simulink library "fm_lib"  (R2014a)
settings: Solver=ode45  SolverMode=SingleTasking  StartTime=0.0  StopTime=10.0  RelTol=1e-3
(part 1 of 2)
Description:
  | PSAT Library
settings Model: ExtModeAutoUpdateStatusClock=off  Creator=fmilano  LastModifiedBy=m.shariatzadeh

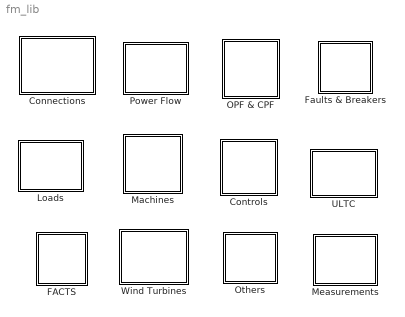
== system fm_lib ==
  Connections : Subsystem  Tag=PSATfolder  Description=Connections  mask(Bus & Connections){}
      mask init:
      | x = fm_draw('connections');
      mask Display: image(x)
  Controls : Subsystem  Tag=PSATfolder  Description=Controls
      mask init:
      | x = fm_draw('controls');
      mask Display: image(x)
  FACTS : Subsystem  Tag=PSATfolder  Description=FACTS
      mask init:
      | x = fm_draw('facts');
      mask Display: image(x)
  Faults & Breakers : Subsystem  Tag=PSATfolder  Description=Switches
      mask init:
      | x = fm_draw('fault');
      mask Display: image(x)
  Loads : Subsystem  Tag=PSATfolder  Description=Loads
      mask init:
      | x = fm_draw('loads');
      mask Display: image(x)
  Machines : Subsystem  Tag=PSATfolder  Description=Machines
      mask init:
      | x = fm_draw('machines');
      mask Display: image(x)
  Measurements : Subsystem  Tag=PSATfolder  Description=Switches
      mask init:
      | x = fm_draw('measures');
      mask Display: image(x)
  OPF & CPF : Subsystem  Tag=PSATfolder  Description=OPFandCPF
      mask init:
      | x = fm_draw('opfcpf');
      mask Display: image(x)
  Others : Subsystem  Tag=PSATfolder  Description=Others
      mask init:
      | x = fm_draw('others');
      mask Display: image(x)
  Power Flow : Subsystem  Tag=PSATfolder  Description=PowerFlow
      mask init:
      | x = fm_draw('powerflow');
      mask Display: image(x)
  ULTC : Subsystem  Tag=PSATfolder  Description=ULTC
      mask init:
      | x = fm_draw('ultc');
      mask Display: image(x)
  Wind Turbines : Subsystem  Tag=PSATfolder  Description=Controls
      mask init:
      | x = fm_draw('wind');
      mask Display: image(x)

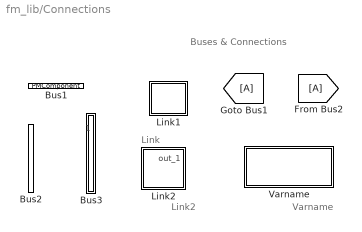
== system fm_lib/Connections ==
  note: Buses & Connections
  note: Link
  note: Link2
  note: Varname
  Bus1 : PMComponent  Tag=PSATblock  Description=Connection  PhysicalDomain=psatdomain  LeftPortType=p1  RightPortType=p1  LConnTagsString=__newl0|__newl1  RConnTagsString=__newr0  mask(Bus){in=2, out=1, p2q=400, p3_4q=[1.00  0.00], p5q=1, p6q=1}
      mask prompts: in "Number of inputs:"; out "Number of outputs:"; p2q "Voltage Rating [kV]"; p3_4q "Voltage initial guess [p.u.  rad]"; p5q "Area number"; p6q "Region number"
      mask help: Bus block.
      mask init:
      | fm_inout
      mask Callback p5q: fm_block
      mask Display: plot([0 1 1 0 0],[0 0 1 1 0])
  Bus2 : PMComponent  Tag=PSATblock  Description=Connection  PhysicalDomain=psatdomain  LeftPortType=p1  RightPortType=p1  LConnTagsString=__newl0|__newl1|__newl2  RConnTagsString=__newr0|__newr1  mask(Bus){in=3, out=2, p2q=400, p3_4q=[1.00   0.00], p5q=1, p6q=1}
      mask prompts: in "Number of inputs:"; out "Number of outputs:"; p2q "Voltage Rating [kV]"; p3_4q "Voltage initial guess [p.u.   rad]"; p5q "Area number"; p6q "Region number"
      mask help: Bus block
      mask init:
      | fm_inout
      mask Callback p5q: fm_block
      mask Display: plot([0 1 1 0 0],[0 0 1 1 0])
  Bus3 : Subsystem  Tag=PSATblock  Description=Connection  mask(Bus){in=3, out=2, p2q=400, p3_4q=[1.00  0.00], p5q=1, p6q=1, ins=0, ous=1}
      mask prompts: in "Number of inputs:"; out "Number of outputs:"; p2q "Voltage Rating [kV]"; p3_4q "Voltage initial guess [p.u.  rad]"; p5q "Area number"; p6q "Region number"; ins "Input Signals"; ous "Output Signals"
      mask help: Bus block.
      mask init:
      | fm_inout
      mask TypeOptions ins: 0 | 1 | 2 | 3
      mask TypeOptions ous: 0 | 1 | 2 | 3
      mask Display: plot([0 1 1 0 0],[0 0 1 1 0])
  Link1 : Subsystem  Tag=PSATblock  Description=Connection  mask(Link){}
      mask help: Link block
      mask init:
      | rot = strcmp(get_param(gcb,'NamePlacement'),'normal');
      mask Display:
      | plot([0.45 0],[0.5 0.5],[1 0.55],[0.5 0.5])
      | color('green')
      | plot([0.45 0.55 0.55 0.45 0.45],[0.45 0.45 0.55 0.55 0.45],[0.5 0.5],rot*0.45+[0.1 0.45])
      | plot([0.45 0.55 0.55 0.45 0.45],rot*0.9+[0 0 0.1 0.1 0],1-rot,1-rot)
  Link2 : Subsystem  Tag=PSATblock  Description=Connection  mask(Link2){}
      mask help: Link block.
      mask Display:
      | plot([0 0.45],[0.5 0.5],[0.5 0.5],[0 0.4],[0.5 1],[0 0])
      | color('green')
      | plot([0.5 0.5],[0.6 1],[0.5 0.9],[1 1])
      | plot([0.9 0.985 0.985 0.9 0.9],[0.1 0.1 -0.1 -0.1 0.1]+1)
      | plot([0.45 0.55 0.55 0.45 0.45],[0.6 0.6 0.4 0.4 0.6])
      | plot(0, -0.5,0,1.5)
  Varname : Subsystem  Tag=PSATblock  Description=OPF & CPF  mask(Varname){pxq=[]}
      mask prompts: pxq "Plot variable list"
      mask help: This block defines the indexes of the variables to be plotted.
      mask Display:
      | plot([-2 22 22 -2 -2],[-1.1 -1.1 1.1 1.1 -1.1])
      | color('blue')
      | text(0,0.1,'Plot variable list')

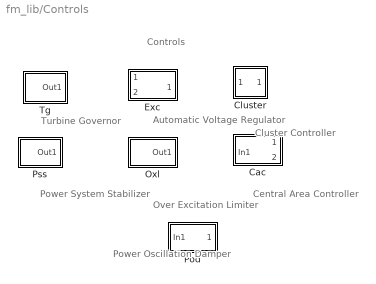
== system fm_lib/Controls ==
  note: Controls
  note: Turbine
      | Governor
  note: Automatic Voltage
      | Regulator
  note: Cluster
      | Controller
  note: Central Area
      | Controller
  note: Over Excitation
      | Limiter
  note: Power System
      | Stabilizer
  note: Power Oscillation
      | Damper
  Cac : Subsystem  Tag=PSATblock  Description=Controls  mask(Cac){p4q=2, p6q=0.02, p7q=1, p8_9q=[1.1  0.9], p10q=on}
      mask prompts: p4q "Number of connected clusters"; p6q "Integral gain constant KI"; p7q "Proportional gain constant KP"; p8_9q "Control signal limits q_max, q_min"; p10q "Connected"
      mask help: This block defines a Central Area Controller
      mask init:
      | fm_inout
      | [x,y] = fm_draw('C');
      mask TypeOptions p4q: 1 | 2 | 3 | 4 | 5 | 6 | 7 | 8 | 9 | 10 | 11 | 12
      mask Callback p10q: fm_block
      mask Display:
      | plot([1 0 0 1 1],[1 1 0 0 1])
      | color('red')
      | plot([0.35 0.5 0.65],[0.2 0.8 0.2],[0.4 0.6],[0.4 0.4])
      | plot(0.1+0.2*x,0.5+0.6*y,0.7+0.2*x,0.5+0.6*y)
  Cluster : Subsystem  Tag=PSATblock  Description=Controls  mask(Cluster){p4q=5, p5q=0, p6q=1, p8_9q=[0.15  -0.2], p10q=on}
      mask prompts: p4q "Integral time constant T [s]"; p5q "Equivalent reactance Xtg [p.u.]"; p6q "Equivalent reactance Xeq [p.u.]"; p8_9q "Output signal limits Vs_max, Vs_min"; p10q "Connected"
      mask help: This block defines Cluster Controler (Secondary Voltage Regulator).
      mask init:
      | [x,y] = fm_draw('C');
      mask Callback p10q: fm_block
      mask Display:
      | plot([1 0 0 1 1],[1 1 0 0 1])
      | color('red')
      | plot(0.1+0.3*x,0.5+0.6*y,0.6+0.3*x,0.5+0.6*y)
  Exc : Subsystem  Tag=PSATblock  Description=Controls  mask(Exc){p2q=1, p3q=5.00, p4q=-5.00, p5q=400, p6q=0.10, p7q=0.45, p8q=1.00, p9q=0.01, p10q=1.00, p11q=0.001, p12_13q=[0.0006  0.9], in=2, p14q=on}
      mask prompts: p2q "Automatic Voltage Regulator Type"; p3q "Maximum Regulator Voltage [p.u.]"; p4q "Minimum Regulator Voltage [p.u.]"; p5q "Regulator Gain m0 [p.u./p.u.]"; p6q "First Regulator Pole T1 [s]"; p7q "First Regulator Zero T2 [s]"; p8q "Second Regulator Pole T3 [s]"; p9q "Second Regulator Zero T4 [s]"; p10q "Time Constant of the Field Circuit Td [s]"; p11q "Time Delay of the Measurement System Tr [s]"; p12_13q "Coefficient of the Ceiling Function (A B)"; in "Number of input signals"; p14q "Connected"
      mask help: This block defines an Automatic Voltage Regulator.
      mask init:
      | fm_inout
      | [x,y] = fm_draw('R');
      mask Help:
      | This block defines an Automatic Voltage Regulator.
      | There are three kind of regulators:
      | 
      | Type 1:
      | 
      |      IEEE Model 1
      | 
      | Type 2:
      | 
      |      IEEE Model 2
      | 
      | Type 3:
      | 
      |      IEEE Model 3
      mask TypeOptions p2q: 1 | 2 | 3
      mask Callback p2q: fm_block
      mask TypeOptions in: 0 | 1 | 2 | 3
      mask Callback p14q: fm_block
      mask Display:
      | plot([-1.8 4.1 4.1 -1.8 -1.8],[-1.5 -1.5 1.5 1.5 -1.5])
      | color('red')
      | plot([-1.3 -0.5],[-1 1],[-0.5 0.3],[1 -1],[-0.9 -0.1],[0.0 0.0])
      | plot(2.8+1.3*x,2*y,1.5+[-1.3 -0.5],[1 -1],1.5+[-0.5 0.3],[-1 1])
  Oxl : Subsystem  Tag=PSATblock  Description=Controls  mask(Oxl){p2q=10, p3q=on, p4q=0.2, p5q=0.18, p6q=2.7, p7q=0.05, p8q=on}
      mask prompts: p2q "Integrator time constant T0 [s]"; p3q "Use generator Xd and Xq"; p4q "d-axis estimated reactance Xd [p.u.]"; p5q "q-axis estimated reactance Xq [p.u.]"; p6q "Maximum Field Current [p.u.]"; p7q "Maximum output signal [p.u.]"; p8q "Connected"
      mask help: This block defines a breaker.
      mask init:
      | [x,y] = fm_draw('O');
      mask Callback p3q: fm_block
      mask Callback p8q: fm_block
      mask Display:
      | plot([-1.8 4.1 4.1 -1.8 -1.8],[-1.5 -1.5 1.5 1.5 -1.5])
      | color('red')
      | plot(1.8+[-1.3 0],[1 -1],1.8+[-1.3 0],[-1 1])
      | plot(1.5*x-1.2,2*y,[2.3 2.3],[1 -1],[2.3 3.6],[-1 -1])
  Pod : Subsystem  Tag=PSATblock  Description=Controls  mask(Pod){p3q=Bus_V, p5_6q=[0.2 -0.2], p7_8q=[-0.1 5], p9_10q=[0.4 0.2], p11_12q=[0.4 0.2], p13q=on}
      mask prompts: p3q "Input signal:"; p5_6q "Vmax and Vmin Stabilizer Output [p.u., p.u.]"; p7_8q "Gain Kw and time constant Tw  [p.u./p.u., s]"; p9_10q "Lead-Lag time constants T1 and T2 [s, s]"; p11_12q "Lead-Lag time constants T3 and T4 [s, s]"; p13q "Connected"
      mask help: This block defines a Suplementary Stabilizing Control Loop.
      mask init:
      | [xP,yP] = fm_draw('P');
      | [xO,yO] = fm_draw('O');
      | [xD,yD] = fm_draw('D');
      mask TypeOptions p3q: Bus_V | Line_P_from_bus | Line_P_to_bus | Line_I_from_bus | Line_I_to_bus | Line_Q_from_bus | Line_Q_to_bus
      mask Callback p3q: fm_block
      mask Callback p13q: fm_block
      mask Display:
      | plot([-1.8 4.8 4.8 -1.8 -1.8],[-1.5 -1.5 1.5 1.5 -1.5])
      | color('red')
      | plot(1.5*xP-0.7,2*yP,0.7+1.5*xO,2*yO,3.5+1.5*xD,2*yD)
  Pss : Subsystem  Tag=PSATblock  Description=Controls  mask(Pss){p2q=4, p3q=omega, p4_5q=[0.05 -0.05], p6_7q=[50  0.5], p14_15q=20  5, p8_9_10_11q=[0.1 0.05 0.01 0.005], p12_13q=[25 0.5], p16_17_18_19q=[0.045  0.045  0.045  -0.045], p20_21q=[1.000  0.95], p22q=off, p23q=on}
      mask prompts: p2q "PSS model"; p3q "Input Signal"; p4_5q "Max and Min Stabilizer Output [p.u.]"; p6_7q "Gain Kw and time constant Tw  [p.u./p.u., s]"; p14_15q "Electrical power gain Kp and voltage gain Kv [p.u./p.u., p.u./p.u.]"; p8_9_10_11q "Lead-Lag time constants T1, T2, T3, T4 [s, s, s, s]"; p12_13q "Gain Ka and time constant Ta [p.u./p.u., s]"; p16_17_18_19q "Additional signal limits Va_max, Va_thr, V3_max and V3_min [p.u., p.u., p.u., p.u.]"; p20_21q "Threshold limits E_thr and w_thr [p.u., p.u.]"; p22q "Allow switch S2"; p23q "Connected"
      mask help: This block defines a Power System Stabilizer.
      mask init:
      | [xs,ys] = fm_draw('S');
      | [xp,yp] = fm_draw('P');
      mask TypeOptions p2q: 1 | 2 | 3 | 4 | 5
      mask Callback p2q: fm_block
      mask TypeOptions p3q: omega | power | voltage
      mask Callback p23q: fm_block
      mask Display:
      | plot([-1.8 4.1 4.1 -1.8 -1.8],[-1.5 -1.5 1.5 1.5 -1.5])
      | color('red')
      | plot(1.5*xp-0.7,2*yp,1.2+1.5*xs,2*ys,2.8+1.5*xs,2*ys)
  Tg : Subsystem  Tag=PSATblock  Description=Controls  mask(Tg){p2q=4, p3q=1.00, p4q=0.2, p5q=1.0, p6q=0.0, p7q=0.10, p8q=-0.10, p9q=0.04, p10q=5.0, p11q=0.04, p12q=0.3, p13q=1.0, p14q=0.5, p15q=1.0, p16q=1.5, p17q=1.0, p18q=1.163, p19q=0.105, p20q=on}
      mask prompts: p2q "Turbine governor type"; p3q "Reference speed [p.u.]"; p4q "Pilot valve droop [p.u./p.u.]"; p5q "Maximum torque [p.u.]"; p6q "Minimum torque [p.u.]"; p7q "Maximum gate opening rate vmax [p.u.]"; p8q "Minimum gate opening rate vmin [p.u.]"; p9q "Pilot valve time constant Tp[s]"; p10q "Dashpot time constant Tr[s]"; p11q "Permanent speed droop sigma[p.u./p.u.]"; p12q "Temporary speed droop delta[p.u./p.u.]"; p13q "Water starting time Tw[s]"; p14q "Patical derivative of turbine flow rate with respect to tubine head a11"; p15q "Patical derivative of turbine flow rate with respect to gate position a13"; p16q "Patical derivative of turbine torque with respect to tubine head a21"; p17q "Patical derivative of turbine torque with respect to gate position a23"; p18q "Proportional droop Kp [p.u./p.u.]"; p19q "Integral droop Ki [p.u./p.u.]"; p20q "Connected"
      mask help: This block defines a Turbine Governor.
      mask init:
      | [x,y] = fm_draw('G');
      mask TypeOptions p2q: 1 | 2 | 3 | 4 | 5 | 6
      mask Callback p2q: fm_block
      mask Callback p20q: fm_block
      mask Display:
      | plot([-1.8 2.8 2.8 -1.8 -1.8],[-1.5 -1.5 1.5 1.5 -1.5])
      | color('red')
      | plot([-0.5 -0.5],[-1 1],[-1.3 0.3],[1 1])
      | plot(1.4+x,y)

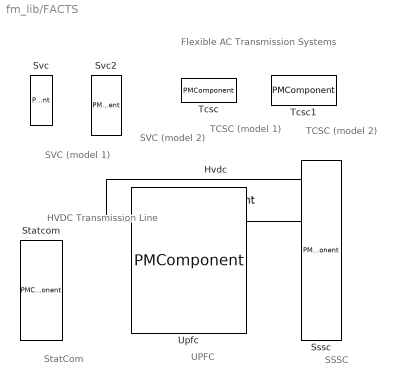
== system fm_lib/FACTS ==
  note: Flexible AC Transmission Systems
  note: TCSC (model 2)
  note: TCSC
      | (model 1)
  note: SVC
      | (model 1)
  note: SVC
      | (model 2)
  note: HVDC
      | Transmission
      | Line
  note: StatCom
  note: UPFC
  note: SSSC
  Hvdc : PMComponent  Tag=PSATblock  Description=FACTS  PhysicalDomain=psatdomain  LeftPortType=p1  RightPortType=p1  LConnTagsString=__newl0  RConnTagsString=__newr0  mask(Hvdc){p3_6q=[1000  60], p4_5q=[400  400], p7_8q=[400  2.5], p9_10q=[0.1345   0.1257], p11_12q=[1.25  1.25], p13_14q=[20  25], p15_16q=[0.0625  0.200], p17_18q=[120  5], p19_20q=[40  18], p21_22_23_24q=[1.0   0.1  0.9  0.0], p25q=Current_control, p26_27_28q=[0.5  0.6  1.0], p29q=on}
      mask prompts: p3_6q "Power and Frequency Ratings [MVA,  Hz]"; p4_5q "Voltage Rating at Terminal Buses [kV, kV]"; p7_8q "DC Ratings (Vn_dc, In_dc) [kV, kA]"; p9_10q "Transformer Reactances (Xcr  Xci) [p.u.  p.u.]"; p11_12q "Tap Ratios (Ar Ai) [p.u./p.u.  p.u./p.u.]"; p13_14q "PI Regulator Constants (Ki, Kp)"; p15_16q "DC Line Parameters (Rdc Ldc) [p.u.  p.u.]"; p17_18q "Rectifier Angle Limits (a_max, a_min) [deg  deg]"; p19_20q "Inverter Angle Limits (g_max, g_min) [deg  deg]"; p21_22_23_24q "Reference Current Limits (I0rmax I0rmin I0imax I0imin) [p.u.]"; p25q "Control type"; p26_27_28q "Current, active power and dc voltage orders [p.u.  p.u.  p.u.]"; p29q "Connected"
      mask help: This block defines a HVDC connection.
      mask init:
      | [x,y] = fm_draw('circle');
      mask TypeOptions p25q: Current_control | Power_control | Voltage_control
      mask Callback p25q: fm_block
      mask Callback p29q: fm_block
      mask Display:
      | plot(0.7+[0 4 4 0 0],[-2 -2 2 2 -2])
      | plot(9.7+[0 4 4 0 0],[-2 -2 2 2 -2])
      | plot([4.7 9.7],[-1.25 -1.25],[4.7 9.7],[1.25 1.25])
      | 
      | plot(x-2,y,x-0.6,y,x+15,y,x+16.4,y)
      | color('green')
      | plot(-2+[-1 -1.3],[0 0],-2+[2.4 2.7],[0 0])
      | plot(-2+[-0.8 0.7],[-1.2 1.2],-2+[0.5 0.7],[1.1 1.2],-2+[0.7 0.7],[1.0 1.2])
      | plot(15+[-1 -1.3],[0 0],15+[2.4 2.7],[0 0])
      | plot(16.4+[-0.8 0.7],[-1.2 1.2],16.4+[0.5 0.7],[1.1 1.2],16.4+[0.7 0.7],[1.0 1.2])
      | 
      | color('magenta')
      | text(1.1,1.2,'R')
      | text(10.1,1.2,'I')
      | plot(0.7+[1 3 2 1],[-0.9 -0.9 0.9 -0.9])
      | plot(9.7+[1 3 2 1],[-0.9 -0.9 0.9 -0.9])
      | plot(0.7+[2 2],[0.9 1.25],0.7+[2 2],[-0.9 -1.25],0.7+[1.2 2.8],[0.9 0.9])
      | plot(9.7+[2 2],[0.9 1.25],9.7+[2 2],[-0.9 -1.25],9.7+[1.2 2.8],[0.9 0.9])
      | plot(0.7+[2 2.5],[0.9 1.25],9.7+[2 2.5],[0.9 1.25])
  Sssc : PMComponent  Tag=PSATblock  Description=FACTS  PhysicalDomain=psatdomain  LeftPortType=p1  RightPortType=p1  LConnTagsString=__newl0  RConnTagsString=__newr0  mask(Sssc){p3_4_5q=[100  230  60], p2q=constant_voltage, p10q=constant_line_power, p6q=25, p7q=0.1, p8_9q=[1.15  0.85], p11_12q=[10 50], p13q=on}
      mask prompts: p3_4_5q "Power, Voltage and Frequency Ratings [MVA, kV, Hz]"; p2q "Operation mode:"; p10q "Scheduling strategy:"; p6q "Percentage of series compensation Cp [%]"; p7q "Regulator time constant Tr [s]"; p8_9q "Max and Min voltage [p.u.  p.u.]"; p11_12q "Porportional and integral gains KP and KI"; p13q "Connected"
      mask help: This block describes a SSSC component.
      mask init:
      | [x,y] = fm_draw('circle');
      | [xc,yc] = fm_draw('cap');
      | [xa,ya] = fm_draw('acdc2');
      mask Help:
      | Tree control methodology are available:
      | 
      | Type 1, Magnitude control: m controls AC voltage by mean of a lead-lag transfer function, whereas alpha controls DC voltage by mean of a PI regulator.
      | 
      | Type 2, Phase control: alpha controls AC voltage by mean of a PI regulator along with a lead-lag transfer function, whereas m is kept at 0.9.
      | 
      | Type 3, Phase control: alpha controls AC voltage by mean of a two poles and one zero transfer function, whereas m is kept at 0.9. In this case parameters Kp and Ki are respectively the gain and the time constant of the low pass filter.
      mask TypeOptions p2q: constant_voltage | constant_reactance | constant_power
      mask Callback p2q: fm_block
      mask TypeOptions p10q: constant_line_power | constant_angle
      mask Callback p13q: fm_block
      mask Display:
      | plot([0.3 0.3 -0.95 -0.95 0.3],[-1.7 2.7 2.7 -1.7 -1.7])
      | plot([-0.75 -0.75 -0.4],[-1.7 -5 -5],[0.1 0.1 -0.25],[-1.7 -5 -5],[-0.4 -0.4],[-4 -6])
      | plot(-0.15+0.1*xc,-5+yc)
      | plot([-0.325 -0.325],[2.7 3.5],[-0.575 -0.95],[5.9 5.9],[-0.075 0.3],[5.9 5.9],0,17.8)
      | plot(0.25*x-0.325,4.5+y,0.25*x-0.325,5.9+y)
      | 
      | color('magenta')
      | plot(xa,ya)
  Statcom : PMComponent  Tag=PSATblock  Description=FACTS  PhysicalDomain=psatdomain  LeftPortType=p1  RightPortType=p1  LConnTagsString=__newl0  mask(Statcom){p2_3_4q=[100  230  60], p5_6q=[50  0.1], p7_8q=[1.2  0.8], p9q=on}
      mask prompts: p2_3_4q "Power, voltage and frequency ratings [MVA, kV, Hz]"; p5_6q "Gain and time constant of the current control Kr, Tr [p.u./p.u.  s]"; p7_8q "Max and Min Current [p.u. p.u.]"; p9q "Connected"
      mask help: This block describes a StatCom component.
      mask init:
      | [x,y] = fm_draw('circle');
      | [xc,yc] = fm_draw('cap');
      | [xa,ya] = fm_draw('acdc2');
      mask Help:
      | Tree control methodology are available:
      | 
      | Type 1, Magnitude control: m controls AC voltage by mean of a lead-lag transfer function, whereas alpha controls DC voltage by mean of a PI regulator.
      | 
      | Type 2, Phase control: alpha controls AC voltage by mean of a PI regulator along with a lead-lag transfer function, whereas m is kept at 0.9.
      | 
      | Type 3, Phase control: alpha controls AC voltage by mean of a two poles and one zero transfer function, whereas m is kept at 0.9. In this case parameters Kp and Ki are respectively the gain and the time constant of the low pass filter.
      mask Callback p9q: fm_block
      mask Display:
      | plot([9.2 4.8 4.8 9.2 9.2],[0.3 0.3 -0.95 -0.95 0.3])
      | plot([9.2 12.5  12.5],[-0.75 -0.75 -0.4],[9.2 12.5  12.5],[0.1 0.1 -0.25],[11.5 13.5],[-0.4 -0.4])
      | plot(12.5-yc,-0.15+0.1*xc)
      | plot([4.8 4],[-0.325 -0.325],[0.6 0],[-0.325 -0.325])
      | plot(3-y,0.25*x-0.325,1.6-y,0.25*x-0.325)
      | color('magenta'), plot(7.5-ya,xa)
  Svc : PMComponent  Tag=PSATblock  Description=FACTS  PhysicalDomain=psatdomain  LeftPortType=p1  RightPortType=p1  LConnTagsString=__newl0  mask(Svc){p2_3_4q=[100   230   60], p5q=1, p6q=10, p7q=100, p8q=1.00, p9_10q=[1.00   -1.00], p11_12q=[0.001  0.000], p13_14q=[1.000  0.01], p15_16q=[0.20   0.10], p17q=on}
      mask prompts: p2_3_4q "Power, Voltage and Frequency Ratings [MVA, kV, Hz]"; p5q "Model Type"; p6q "Regulator Time Constant Tr [s]"; p7q "Regulator Gain Kr [p.u./p.u.]"; p8q "Reference Voltage [p.u.]"; p9_10q "B_max and B_min [p.u.  p.u.]"; p11_12q "Integral deviation Kd and transient time constant T1 [p.u. s]"; p13_14q "Measurement gain and time delay Km, Tm [p.u. s]"; p15_16q "Inductive and capacitive reactances Xl and Xc [p.u. p.u.]"; p17q "Connected"
      mask help: This block describes an SVC component.
      mask init:
      | [xi,yi] = fm_draw('ind');
      | [xc,yc] = fm_draw('cap');
      | [xa,ya] = fm_draw('acdc');
      mask TypeOptions p5q: 1 | 2
      mask Callback p5q: fm_block
      mask Callback p17q: fm_block
      mask Display: plot([1 0.8],[0.5 0.5],[0 0.2],[0.5 0.5],[0.8 0.8 0.2 0.2 0.8],[0 1 1 0 0]), plot([1 1],[-0.1 1.1],[1.05 1.05],[0.1 0.9],[1.1 1.1],[0.3 0.7]), color('green'), plot([0.1 0.3 0.7 0.9],[-0.4 -0.4 1.4 1.4])
  Svc2 : PMComponent  Tag=PSATblock  Description=FACTS  PhysicalDomain=psatdomain  LeftPortType=p1  RightPortType=p1  LConnTagsString=__newl0  mask(Svc){p2_3_4q=[100   230   60], p5q=2, p6q=10, p7q=100, p8q=1.00, p9_10q=[1.00   -1.00], p11_12q=[0.001  0.000], p13_14q=[1.000  0.01], p15_16q=[0.20   0.10], p17q=on}
      mask prompts: p2_3_4q "Power, Voltage and Frequency Ratings [MVA, kV, Hz]"; p5q "Model Type"; p6q "Regulator Time Constant T2 [s]"; p7q "Regulator Gain K [p.u./p.u.]"; p8q "Reference Voltage [p.u.]"; p9_10q "Alpha_max and Alpha_min [rad rad]"; p11_12q "Integral deviation Kd and transient time constant T1 [p.u. s]"; p13_14q "Measurement gain and time delay Km, Tm [p.u. s]"; p15_16q "Inductive and capacitive reactances Xl and Xc [p.u. p.u.]"; p17q "Connected"
      mask help: This block describes an SVC component.
      mask init:
      | [xi,yi] = fm_draw('ind');
      | [xc,yc] = fm_draw('cap');
      | [xa,ya] = fm_draw('acdc');
      mask TypeOptions p5q: 1 | 2
      mask Callback p5q: fm_block
      mask Display: plot([-1.6 -1.8 -1.8],[0.5 0.5 4],[0.2 0.2],[0.5 4],[-0.9 -0.9],[3 5],[0 0.2],[0.5 0.5],[-0.65 -0.85],[0.5 0.5],[-1.8 -0.9],[4 4],[0.2 -0.8],[4 4],[0.2 0.4],[1.9 1.9],[-1.8 -2],[1.9 1.9],[0.4 0.4],[2.9 0.9],[0.5 0.5],[2.5 1.3],[0.6 0.6],[2.1 1.7]), plot(-0.7+0.1*xc,4+yc,-1.15+0.175+0.125*yi,0.5+0.5*xi,-1.15-0.325+0.125*yi,0.5+0.5*xi,-1.15-0.075+0.125*yi,0.5+0.5*xi), color('magenta'), plot(xa,ya)
  Tcsc : PMComponent  Tag=PSATblock  Description=FACTS  PhysicalDomain=psatdomain  LeftPortType=p1  RightPortType=p1  LConnTagsString=__newl0  RConnTagsString=__newr0  mask(Tcsc){p5_6_7q=[100   230   60], p2q=Xc, p3q=constant_power_flow, p4q=constant_line_power, p8q=10, p9q=0.5, p10_11q=[0.5   -0.5 ], p12_13q=[5 1], p14_15q=[0.2  0.1], p16q=10, p17q=on}
      mask prompts: p5_6_7q "Power, Voltage and Frequency Ratings [MVA, kV, Hz]"; p2q "Model type:"; p3q "Operation mode:"; p4q "Scheduling strategy:"; p8q "Percentage of series compensation [%]"; p9q "Regulator time constant Tr [s]"; p10_11q "Xc_max and Xc_min [p.u.  p.u.]"; p12_13q "Proportional and Integral gains Kp and Ki"; p14_15q "XL and XC [p.u.  p.u.]"; p16q "Gain for stabilizing signal Kr [p.u./p.u.]"; p17q "Connected"
      mask help: This block describes a TCSC component.
      mask init:
      | [xi,yi] = fm_draw('ind');
      | [xc,yc] = fm_draw('cap');
      | [xa,ya] = fm_draw('acdc');
      mask TypeOptions p2q: Xc | Alpha
      mask Callback p2q: fm_block
      mask TypeOptions p3q: constant_admittance | constant_power_flow
      mask TypeOptions p4q: constant_line_power | constant_angle
      mask Callback p17q: fm_block
      mask Display: plot([1 0.8],[0.5 0.5],[0 0.2],[0.5 0.5],[0.8 0.8 0.2 0.2 0.8],[0 1 1 0 0]), color('green'), plot([0.1 0.3 0.7 0.9],[-0.4 -0.4 1.4 1.4])
  Tcsc1 : PMComponent  Tag=PSATblock  Description=FACTS  PhysicalDomain=psatdomain  LeftPortType=p1  RightPortType=p1  LConnTagsString=__newl0  RConnTagsString=__newr0  mask(Tcsc){p5_6_7q=[100   230   60], p2q=Alpha, p3q=constant_power_flow, p4q=constant_line_power, p8q=10, p9q=0.5, p10_11q=[0.5   -0.5 ], p12_13q=[5 1], p14_15q=[0.2  0.1], p16q=10, p17q=on}
      mask prompts: p5_6_7q "Power, Voltage and Frequency Ratings [MVA, kV, Hz]"; p2q "Model type:"; p3q "Operation mode:"; p4q "Scheduling strategy:"; p8q "Percentage of series compensation [%]"; p9q "Regulator time constant Tr [s]"; p10_11q "Alpha_max and Alpha_min [rad  rad]"; p12_13q "Proportional and Integral gains Kp and Ki"; p14_15q "XL and XC [p.u.  p.u.]"; p16q "Gain for stabilizing signal Kr [p.u./p.u.]"; p17q "Connected"
      mask help: This block describes a TCSC component.
      mask init:
      | [xi,yi] = fm_draw('ind');
      | [xc,yc] = fm_draw('cap');
      | [xa,ya] = fm_draw('acdc');
      mask TypeOptions p2q: Xc | Alpha
      mask Callback p2q: fm_block
      mask TypeOptions p3q: constant_admittance | constant_power_flow
      mask TypeOptions p4q: constant_line_power | constant_angle
      mask Callback p17q: fm_block
      mask Display:
      | plot([-1.6 -1.8 -1.8],[0.5 0.5 4],[0.2 0.2],[0.5 4],[-0.9 -0.9],[3 5],[0 0.2],[0.5 0.5],[-0.65 -0.85],[0.5 0.5],[-1.8 -0.9],[4 4],[0.2 -0.8],[4 4],[0.2 0.4],[1.9 1.9],[-1.8 -2],[1.9 1.9]), plot(-0.7+0.1*xc,4+yc,-1.15+0.175+0.125*yi,0.5+0.5*xi,-1.15-0.325+0.125*yi,0.5+0.5*xi,-1.15-0.075+0.125*yi,0.5+0.5*xi),
      | color('magenta'), plot(xa,ya)
  Upfc : PMComponent  Tag=PSATblock  Description=FACTS  PhysicalDomain=psatdomain  LeftPortType=p1  RightPortType=p1  LConnTagsString=__newl0  RConnTagsString=__newr0  mask(Upfc){p3_4_5q=[100  230  60], p2q=constant_voltage, p6q=25, p7_8q=[50 0.1], p9_10q=[1.15 0.85], p11_12q=[1.15 0.85], p13_14q=[1.1 0.9], p15q=on, p16q=on, p17q=on, p18q=on}
      mask prompts: p3_4_5q "Power, Voltage and Frequency Ratings [MVA, kV, Hz]"; p2q "Operation mode:"; p6q "Percentage of series compensation Cp [%]"; p7_8q "Gain and time constant Kr and Tr [p.u./p.u. s]"; p9_10q "Max and min Vp [p.u. p.u.]"; p11_12q "Max and min Vq [p.u. p.u.]"; p13_14q "Max and min Iq [p.u. p.u.]"; p15q "Stabilizing Vp signal (series voltage)"; p16q "Stabilizing Vq signal (quadrature voltage)"; p17q "Stabilizing Iq signal (quadrature current)"; p18q "Connected"
      mask help: This block describes a UPFC component.
      mask init:
      | [x,y] = fm_draw('circle');
      | [xc,yc] = fm_draw('ind');
      | [xa,ya] = fm_draw('acdc2');
      mask Help:
      | Tree control methodology are available:
      | 
      | Type 1, Magnitude control: m controls AC voltage by mean of a lead-lag transfer function, whereas alpha controls DC voltage by mean of a PI regulator.
      | 
      | Type 2, Phase control: alpha controls AC voltage by mean of a PI regulator along with a lead-lag transfer function, whereas m is kept at 0.9.
      | 
      | Type 3, Phase control: alpha controls AC voltage by mean of a two poles and one zero transfer function, whereas m is kept at 0.9. In this case parameters Kp and Ki are respectively the gain and the time constant of the low pass filter.
      mask TypeOptions p2q: constant_voltage | constant_reactance
      mask Callback p18q: fm_block
      mask Display:
      | plot([0.3 0.3 -0.95 -0.95 0.3],[-1.7 2.7 2.7 -1.7 -1.7])
      | plot(-2+[0.3 0.3 -0.95 -0.95 0.3],[-1.7 2.7 2.7 -1.7 -1.7])
      | plot([-2.325 -2.325],[2.7 3.5],[-2.325 -2.325],[6.9 7.5])
      | plot(0.25*x-2.325,4.5+y,0.25*x-2.325,5.9+y)
      | plot([-0.325 -0.325],[2.7 5.1],[-0.575 -2.95],[7.5 7.5],[-0.075 0.3],[7.5 7.5],0,16.7)
      | plot(0.25*x-0.325,6.1+y,0.25*x-0.325,7.5+y)
      | plot([-0.95 -1.7],[2.2 2.2],[-0.95 -1.7],[-1.2 -1.2])
      | plot([-1.325+0.175  -1.325-0.175],[0.75 0.75],[-1.325 -1.325],[2.2 0.75],[-1.325 -1.325],[0.35 -1.2])
      | plot(-1.325+0.175*yc,0.1+0.25*xc)
      | 
      | color('magenta')
      | plot(xa,ya)
      | plot(xa-2,ya)

== system fm_lib/Faults & Breakers ==
  note: Faults & Operations
  note: Breaker
  note: Fault
  Breaker : PMComponent  Tag=PSATblock  Description=Faults & Breakers  PhysicalDomain=psatdomain  LeftPortType=p1  RightPortType=p1  LConnTagsString=__newl0  RConnTagsString=__newr0  mask(Breaker){p3_4_5q=[100  400  60], p6q=on, p7q=0.00, p8q=0.00, p9q=on, p10q=on}
      mask prompts: p3_4_5q "Power, Voltage and Frequency Ratings [MVA, kV, Hz]"; p6q "Initially close"; p7q "First intervention time [s]"; p8q "Second intervention time [s]"; p9q "Apply first intervention"; p10q "Apply second intervention"
      mask help: This block defines a transmission line breaker.
      mask Callback p6q: fm_block
      mask Display: plot([1 2 2 1 1],[-1 -1 1 1 -1]),color('red'),plot([1 2],[-1 1],[2 1],[-1 1])
  Fault : PMComponent  Tag=PSATblock  Description=Faults & Breakers  PhysicalDomain=psatdomain  LeftPortType=p1  RightPortType=p1  LConnTagsString=__newl0  mask(Fault){p2_3_4q=[100  400  60], p5q=0.00, p6q=0.250, p7q=1e-3, p8q=1e-3}
      mask prompts: p2_3_4q "Power, Voltage and Frequency Ratings [MVA, kV, Hz]"; p5q "Fault Time [s]"; p6q "Fault Clearing Time [s]"; p7q "Fault Resistance [p.u.]"; p8q "Fault Reactance [p.u.]"
      mask help: This block defines a three phase fault.
      mask Display:
      | plot([-2 2],[1 1])
      | color('yellow')
      | plot([1 -1],[1 -0.2],[-1 1],[-0.2 0.2],[1 -1],[0.2 -1],[-1 -1],[-1 -0.7],[-1 -0.2],[-1 -0.8])

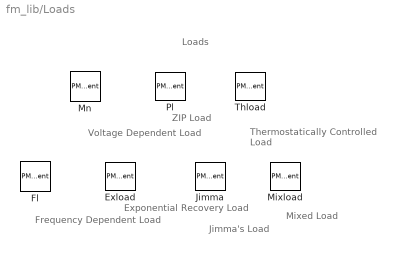
== system fm_lib/Loads ==
  note: Loads
  note: Voltage
      | Dependent
      | Load
  note: ZIP Load
  note: Thermostatically
      | Controlled
      | Load
  note: Frequency
      | Dependent
      | Load
  note: Exponential
      | Recovery
      | Load
  note: Jimma's
      | Load
  note: Mixed
      | Load
  Exload : PMComponent  Tag=PSATblock  Description=Loads  PhysicalDomain=psatdomain  LeftPortType=p1  RightPortType=p1  LConnTagsString=__newl0  mask(Exload){p2q=100, p3_4q=[100 100], p5_6q=[1  1], p7_8q=[2   1.5], p9_10q=[2  1.5], p11q=on}
      mask prompts: p2q "Power ratings [MVA]"; p3_4q "Active and reactive power percentages [%, %]"; p5_6q "Time constants for the real and reactive power dynamics Tp, Tq [s, s]"; p7_8q "Real power exponents Alpha_S, Alpha_T"; p9_10q "Reactive power exponents Beta_S, Beta_T"; p11q "Connected"
      mask help: This block defines Exponential Recovery Loads.
      mask init:
      | [x,y] = fm_draw('R');
      mask Callback p11q: fm_block
      mask Display:
      | plot([1 0 0 1 1],[1 1 0 0 1])
      | color('blue')
      | plot(0.7+0.3*x,0.6*y+0.5,[0.4 0.1 0.1 0.4],[0.8 0.8 0.2 0.2],[0.1 0.25],[0.5 0.5])
  Fl : PMComponent  Tag=PSATblock  Description=Loads  PhysicalDomain=psatdomain  LeftPortType=p1  RightPortType=p1  LConnTagsString=__newl0  mask(Fl){p2q=100, p3_4q=[2  0], p5q=100, p6_7q=[2  0], p8q=0.01, p9q=on}
      mask prompts: p2q "Active power percentage Kp [%]"; p3_4q "Active power voltage and frequency exponents ap, bp"; p5q "Reactive power percentage Kq [%]"; p6_7q "Reactive power voltage and frequency exponents aq, bq"; p8q "Frequency filter time constant Tf [s]"; p9q "Connected"
      mask help:
      | This block defines a general exponential voltage
      | frequency dependent load
      mask Callback p9q: fm_block
      mask Display:
      | plot([-1 -1 1 1 -1],[-1 1 1 -1 -1])
      | color('blue')
      | plot([-0.2 -0.15 0 0 0.15 0.2],[-0.45 -0.5 -0.4 0.35 0.45 0.35],[-0.1 0.15],[0.05 0.05])
  Jimma : PMComponent  Tag=PSATblock  Description=Loads  PhysicalDomain=psatdomain  LeftPortType=p1  RightPortType=p1  LConnTagsString=__newl0  mask(Jimma){p2_3_4q=[100  230  60], p6_7_8q=[33 33 34], p9_10_11q=[33 33 34], p5q=0.01, p12q=100, p13q=on}
      mask prompts: p2_3_4q "Power, voltage and frequency ratings [MVA, kV, Hz]"; p6_7_8q "Percentage of resistance, active current and active power [% % %]"; p9_10_11q "Percentage of reactance, reactive current and reactive power [% % %]"; p5q "High-pass filter time constant Tf [s]"; p12q "Coefficient of voltage time derivative KV [1/s]"; p13q "Connected"
      mask help: This block defines a Jimma's Load.
      mask init:
      | [x,y] = fm_draw('J');
      mask Callback p13q: fm_block
      mask Display:
      | plot([-1 -1 1 1 -1],[-1 1 1 -1 -1]);
      | color('blue')
      | plot(x,y)
  Mixload : PMComponent  Tag=PSATblock  Description=Loads  PhysicalDomain=psatdomain  LeftPortType=p1  RightPortType=p1  LConnTagsString=__newl0  mask(Mixload){p2_3_4q=[100  230  60], p6_10q=[100 100], p5_9q=[0  0], p7_11q=[0  0], p8_12q=[0.1  0.1], p13_14q=[0.01  0.01], p15q=on}
      mask prompts: p2_3_4q "Power, voltage and frequency ratings [MVA, kV, Hz]"; p6_10q "Percentage of active and reactive power Kpv and Kqv [% %]"; p5_9q "Frequency coefficients Kpf and Kqf"; p7_11q "Voltage exponents alpha and beta"; p8_12q "Time constant of dV/dt Tpv and Tqv [s s]"; p13_14q "Filter time constants Tfv and Tft [s s]"; p15q "Connected"
      mask help: This block defines a mixed load.
      mask Callback p15q: fm_block
      mask Display:
      | plot([-1 -1 2.4 2.4 -1],[-1 1 1 -1 -1])
      | color('blue')
      | plot([-0.35 -0.35 0 0.35 0.35],[-0.35 0.35 0.05 0.35 -0.35])
      | plot([0.7 0.7],[-0.35 0.35])
      | plot([1.05 1.75],[-0.35 0.35],[1.05 1.75],[0.35 -0.35])
  Mn : PMComponent  Tag=PSATblock  Description=Loads  PhysicalDomain=psatdomain  LeftPortType=p1  RightPortType=p1  LConnTagsString=__newl0  mask(Mn){p2_3q=[100 400], p4_5q=[80  60], p6_7q=[2.00 2.00], p8q=on, p9q=on}
      mask prompts: p2_3q "Power and voltage ratings [MVA, kV]"; p4_5q "Percentage of active and reactive powers [%, %]"; p6_7q "Voltage exponents for the active and reactive powers"; p8q "Initialize after power flow"; p9q "Connected"
      mask help: This block defines a general exponential voltage load.
      mask Callback p8q: fm_block
      mask Callback p9q: fm_block
      mask Display:
      | plot([-1 -1 1 1 -1],[-1 1 1 -1 -1])
      | color('blue')
      | plot([-0.35 -0.35 0 0.35 0.35],[-0.35 0.35 0.05 0.35 -0.35])
  Pl : PMComponent  Tag=PSATblock  Description=Loads  PhysicalDomain=psatdomain  LeftPortType=p1  RightPortType=p1  LConnTagsString=__newl0  mask(Pl){p2_3_4q=[100 400 60], p5_6_7q=[33 33 33], p8_9_10q=[33 33 33], p11q=on, p12q=on}
      mask prompts: p2_3_4q "Power, voltage and frequency ratings [MVA, kV, Hz]"; p5_6_7q "Percentage of resistance, active current and active power [%, %, %]"; p8_9_10q "Percentage of reactance, reactive current and reactive power [%, %, %]"; p11q "Initialize after power flow"; p12q "Connected"
      mask help: This block defines a ZIP load.
      mask Callback p11q: fm_block
      mask Callback p12q: fm_block
      mask Display:
      | plot([-1 -1 1 1 -1],[-1 1 1 -1 -1])
      | color('blue')
      | plot([0 0],[-0.3 0.3],[-0.3 -0.7 -0.3 -0.7],[-0.3 -0.3 0.3 0.3])
      | plot([0.3 0.3 0.6 0.7 0.7 0.6 0.3],[-0.3 0.3 0.3 0.2 0.1 0 0])
  Thload : PMComponent  Tag=PSATblock  Description=Loads  PhysicalDomain=psatdomain  LeftPortType=p1  RightPortType=p1  LConnTagsString=__newl0  mask(Thload){p2q=50, p3q=100, p4q=25, p5q=10, p6q=1200, p7q=10, p8q=70, p11q=2, p12q=on}
      mask prompts: p2q "% of load to be used as thermostatically controlled load [%]"; p3q "Gain of proportional controller Kp"; p4q "Gain of integral controller Ki"; p5q "Time constant of integral controller Ti [s]"; p6q "Thermostatically controlled load time constant T1 [s]"; p7q "Ambient temperature Ta [F]"; p8q "Reference temperature Tref [F]"; p11q "Ceiling conductance ouput KL"; p12q "Connected"
      mask help: This block defines a thermostatically controlled load
      mask Callback p12q: fm_block
      mask Display:
      | plot([-1 -1 1 1 -1],[-1 1 1 -1 -1])
      | color('blue')
      | plot([-0.5 -0.5 -0.25 -0.25 -0.5],[0.4 0.15 0.15 0.4 0.4])
      | plot([-0.05 -0.05 0.5],[-0.4 0.4 0.4],[-0.05 0.3],[0.05 0.05])

== system fm_lib/Machines ==
  note: Electrical Machines
  note: Synchronous
      | Machine
  note: Induction
      | Machine
  Ind : PMComponent  Tag=PSATblock  Description=Machines  PhysicalDomain=psatdomain  LeftPortType=p1  RightPortType=p1  LConnTagsString=__newl0  mask(Ind){p2_3_4q=[100   25   60], p5q=3, p6q=off, p7q=0.01, p8q=0.15, p9_10q=[0.05  0.15], p11_12q=[0.001  0.04], p13q=5.00, p14q=3.00, p15_16_17q=[1.00  0.00  0.00], p18q=0, p19q=off, p20q=on}
      mask prompts: p2_3_4q "Power, Voltage and Frequency Ratings [MVA, kV, Hz]"; p5q "Dynamic Order"; p6q "Start up"; p7q "Stator Resistance Rs [p.u.]"; p8q "Stator Reactance Xs [p.u.]"; p9_10q "First Cage Resitance Rr1 and Reactance  Xr1 [p.u. p.u.]"; p11_12q "Second Cage Resistance Rr2 and Reactance Xr2 [p.u.  p.u.]"; p13q "Magnetization Reactance Xm [p.u.]"; p14q "Inertia Constant Hm [kWs/kVA]"; p15_16_17q "Mechanical Torque coefficients [a, b, c] [p.u.  p.u.  p.u.]"; p18q "Start up time"; p19q "Allow working as brake"; p20q "Connected"
      mask help:
      | This block defines an asynchronous machine.
      |
      | Order 1:  mechanical equation
      | Order 3:  single cage
      | Order 5:  double cage
      mask init:
      | [x,y] = fm_draw('circle');
      | [xs,ys] = fm_draw('sinus');
      mask TypeOptions p5q: 1 | 3 | 5
      mask Callback p5q: fm_block
      mask Callback p20q: fm_block
      mask Display:
      | plot(x+1.4,y,0.12*xs+1,0.15*ys-0.6)
      | color('blue')
      | plot([1 1 1.4 1.8 1.8],[-0.05 0.7 0.4 0.7 -0.05])
  Syn : Subsystem  Tag=PSATblock  Description=Machines  mask(Syn){p2_3_4q=[370  20   50], p5q=6, p7_6q=[0.001  0.05], p8_9_10q=[1.90  0.302  0.204], p11_12q=[8.00  0.04], p13_14_15q=[1.70  0.50  0.30], p16_17q=[0.80  0.02], p18_19q=[10.00  0.00], p20_21q=[0.00  0.00], p22_23q=[1.00  1.00], p24q=0.002, p25_26q=[0 0], in=0, p27q=1, p28q=on}
      mask prompts: p2_3_4q "Power, voltage and frequency ratings [MVA, kV, Hz]"; p5q "Machine Dynamic Order"; p7_6q "resistance ra and leakage reactance xl [p.u. p.u.]"; p8_9_10q "d-axis reactances Xd, X'd X"d [p.u.,p.u.,p.u.]"; p11_12q "d-axis open circuit time constants T'd0 and T"d0 [s, s]"; p13_14_15q "q-axis reactances Xq, X'q, X"q [p.u.  p.u.  p.u.]"; p16_17q "q-axis open circuit time constants T'q0 and T"q0 [s s]"; p18_19q "Inertia (M = 2H) and Damping [s, p.u.]"; p20_21q "Speed and active power additional signals Kw and Kp [p.u., p.u.]"; p22_23q "Percentage of active and reactive powers at bus [p.u. p.u.]"; p24q "d-axis additional circuit leakage time constant Taa [s]"; p25_26q "Saturation coefficients S(1.0) and S(1.2)"; in "Number of input signals"; p27q "COI number"; p28q "Connected"
      mask help: This block defines a fourth order synchronous machine.
      mask init:
      | fm_inout
      | [x,y] = fm_draw('circle');
      | [xg,yg] = fm_draw('G');
      | [xs,ys] = fm_draw('sinus');
      mask TypeOptions p5q: 8 | 6 | 5.3 | 5.2 | 5.1 | 4 | 3 | 2
      mask Callback p5q: fm_block
      mask TypeOptions in: 0 | 1 | 2
      mask Callback p28q: fm_block
      mask Display:
      | plot(x+1.4,y,0.12*xs+1,0.15*ys-0.6)
      | color('blue')
      | plot(1.4+0.45*xg,0.3+0.45*yg)

== system fm_lib/Measurements ==
  note: Measurements
  note: Bus Frequency
      | Measurement
  note: Phasor
      | Measument Unit
  Busfreq : PMComponent  Tag=PSATblock  Description=Measurements  PhysicalDomain=psatdomain  LeftPortType=p1  RightPortType=p1  LConnTagsString=__newl0  mask(Busfreq){p2q=0.001, p3q=0.001, p4q=on}
      mask prompts: p2q "Frequency deviation filter time constant Tf [s]"; p3q "Frequency filter time constant Tw [s]"; p4q "Connected"
      mask help: This block defines a bus frequency measurement.
      mask Callback p4q: fm_block
      mask Display:
      | plot([-1 0 1 0 -1],[0 1 0 -1 0])
      | color('yellow')
      | plot([-0.2 -0.15 0 0 0.15 0.2],[-0.45 -0.5 -0.4 0.35 0.45 0.35],[-0.1 0.15],[0.05 0.05])
  Pmu : PMComponent  Tag=PSATblock  Description=Measurements  PhysicalDomain=psatdomain  LeftPortType=p1  RightPortType=p1  LConnTagsString=__newl0  mask(Pmu){p2_3q=[230 60], p4q=0.05, p5q=0.05, p6q=on}
      mask prompts: p2_3q "Voltage and frequency rates [kV Hz]"; p4q "Time constant of the voltage magnitude filter [s]"; p5q "Time constant of the voltage phase filter [s]"; p6q "Connected"
      mask help: This block defines a phasor measurement unit (PMU).
      mask init:
      | [xp,yp] = fm_draw('P');
      | [xu,yu] = fm_draw('U');
      | [xm,ym] = fm_draw('M');
      mask Callback p6q: fm_block
      mask Display:
      | plot([-1 0  4 5  4 0 -1],[0 1 1 0 -1 -1 0])
      | color('yellow')
      | plot(xp+0.5,yp,xu+3,yu,xm+2,ym)

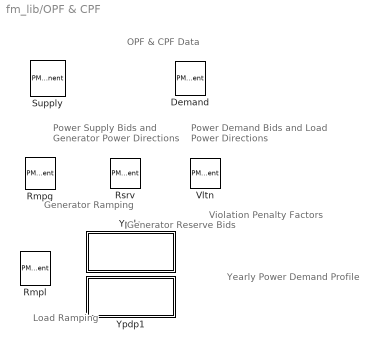
== system fm_lib/OPF & CPF ==
  note: OPF & CPF Data
  note: Power Supply Bids
      | and Generator Power
      | Directions
  note: Power Demand Bids
      | and Load Power
      | Directions
  note: Generator
      | Ramping
  note: Load Ramping
  note: Violation
      | Penalty Factors
  note: Generator
      | Reserve Bids
  note: Yearly Power
      | Demand Profile
  Demand : PMComponent  Tag=PSATblock  Description=OPF & CPF  PhysicalDomain=psatdomain  LeftPortType=p1  RightPortType=p1  LConnTagsString=__newl0  mask(Demand){p2q=100, p3q=0.80, p4q=0.60, p5_6q=[1.00  0.00], p8_9_10q=[0.00  10.5  0.00], p11_12_13q=[0.00  0.00  0.00], p14q=off, p15q=0, p16_17q=[0 0], out=0, p18q=on}
      mask prompts: p2q "Power Rating [MVA]"; p3q "Active Power [p.u.]"; p4q "Reactive Power [p.u.]"; p5_6q "Max and Min Power Demand [p.u.  p.u.]"; p8_9_10q "Cost = a + b*P + c*P^2 [$/h, $/MWh, $/(MW)^2 h]"; p11_12_13q "Cost = a + b*Q + c*Q^2 [$/h, $/MVArh, $/(MVAr)^2 h]"; p14q "Allow Unit Commitment"; p15q "Tie Breaking Cost [$/h]"; p16_17q "Up and down congestion costs [$/h $/h]"; out "Number of Output Signals"; p18q "Connected"
      mask help: This block defines a constant power load for bifurcation and market studies.
      mask init:
      | fm_inout;
      | [xs,ys]=fm_draw('$');
      mask TypeOptions out: 0 | 1
      mask Callback p18q: fm_block
      mask Display:
      | plot([ 1.0000    -0.5   -0.5  1],[ 0    0.866    -0.866    0])
      | color('blue')
      | plot(0.6*xs,0.6*ys)
  Rmpg : PMComponent  Tag=PSATblock  Description=OPF & CPF  PhysicalDomain=psatdomain  LeftPortType=p1  RightPortType=p1  RConnTagsString=__newr0  mask(Rmpg){p2q=100, p3_4q=[1.00  1.00], p5_6q=[1 1], p7_8q=[0 2], p9q=10, p10q=on}
      mask prompts: p2q "Power Rating [MVA]"; p3_4q "Ramp Up and Down Rates [p.u./h  p.u./h]"; p5_6q "Minimum Up and Down Times [h  h]"; p7_8q "Numbers of period up and down at initial time [h  h]"; p9q "Start Up Cost [$]"; p10q "Conneted"
      mask help: This block defines ramping parameters for generators for market studies.
      mask init:
      | [x,y] = fm_draw('circle');
      | [xr,yr] = fm_draw('ramp');
      mask Callback p10q: fm_block
      mask Display:
      | plot(x,y)
      | color('blue')
      | plot(xr,yr)
  Rmpl : PMComponent  Tag=PSATblock  Description=OPF & CPF  PhysicalDomain=psatdomain  LeftPortType=p1  RightPortType=p1  LConnTagsString=__newl0  mask(Rmpl){p2q=100, p3_4q=[1.00  1.00], p5_6q=[1 1], p7_8q=[0 2], p9q=on}
      mask prompts: p2q "Power Rating [MVA]"; p3_4q "Ramp Up and Down Rates  [p.u./h  p.u./h]"; p5_6q "Minimum Up and Down Times [h  h]"; p7_8q "Number of period up and down at initial time [h  h]"; p9q "Connected"
      mask help: This block defines ramping parameters for loads for market studies.
      mask init:
      | [xr,yr] = fm_draw('ramp');
      mask Callback p9q: fm_block
      mask Display:
      | plot([ 1.0000    -0.5   -0.5  1],[ 0    0.866    -0.866    0])
      | color('blue')
      | plot(0.7*xr, 0.6*yr)
  Rsrv : PMComponent  Tag=PSATblock  Description=OPF & CPF  PhysicalDomain=psatdomain  LeftPortType=p1  RightPortType=p1  RConnTagsString=__newr0  mask(Rsrv){p2q=100, p3_4q=0.08   0.00, p5q=10.00, p6q=on}
      mask prompts: p2q "Power Rating [MVA]"; p3_4q "Maximum and Minimum reserve Offer [p.u.  p.u.]"; p5q "Reserve Offer Price [$/MWh]"; p6q "Connected"
      mask help: This block defines generator reserve data.
      mask init:
      | [x,y] = fm_draw('circle');
      | [xr,yr] = fm_draw('R');
      mask Callback p6q: fm_block
      mask Display:
      | plot(x,y)
      | color('blue')
      | plot(0.5*xr,yr)
  Supply : PMComponent  Tag=PSATblock  Description=OPF & CPF  PhysicalDomain=psatdomain  LeftPortType=p1  RightPortType=p1  RConnTagsString=__newr0  mask(Supply){p2q=100, p3q=0.80, p4_5q=[1.00 0.00], p7_8_9q=[0.00  8.80  0.00], p10_11_12q=[0.00  0.00  0.00], p13q=off, p14q=0, p15q=1, p16_17q=[0  0], p18_19q=[0 0], in=0, p20q=on}
      mask prompts: p2q "Power Rating [MVA]"; p3q "Active Power [p.u.]"; p4_5q "Max and Min Power Supply [p.u.  p.u.]"; p7_8_9q "Cost = a + b*P + c*P^2 [$/h, $/MWh, $/(MW)^2 h]"; p10_11_12q "Cost = a + b*Q + c*Q^2 [$/h, $/MVArh, $/(MVAr)^2 h]"; p13q "Allow Unit Commitment"; p14q "Tie Breaking Cost [$/h]"; p15q "Loss participation factor"; p16_17q "Reactive power limits Qmax and Qmin [p.u. p.u.]"; p18_19q "Up and down congestion costs [$/h $/h]"; in "Number of Input Signals"; p20q "Connected"
      mask help: This block defines a PV bus for bifurcation and market studies:
      mask init:
      | fm_inout;
      | [x,y] = fm_draw('circle');
      | [xs,ys] = fm_draw('$');
      mask TypeOptions in: 0 | 1 | 2
      mask Callback p20q: fm_block
      mask Display:
      | plot(x,y)
      | color('blue')
      | plot(xs,ys)
  Vltn : PMComponent  Tag=PSATblock  Description=OPF & CPF  PhysicalDomain=psatdomain  LeftPortType=p1  RightPortType=p1  RConnTagsString=__newr0  mask(Vltn){p2q=100, p3q=0.01, p4q=0.01, p5q=0.01, p6q=0.01, p7q=0.01, p8q=0.01, p9q=0.01, p10q=on}
      mask prompts: p2q "Power Rating [MVA]"; p3q "Deficit Generation Penalty"; p4q "Surplus Generation Penalty"; p5q "Deficit 10 Minutes Reserve Penalty"; p6q "Deficit Synch 10 Min Reserve Penalty"; p7q "Deficit Total Reserve Penalty"; p8q "Surplus Intertie Penalty"; p9q "Deficit Intertie Penalty"; p10q "Connected"
      mask help: This block defines penalty factors for generators for market studies.
      mask init:
      | [x,y] = fm_draw('circle');
      mask Callback p10q: fm_block
      mask Display:
      | plot(x,y)
      | color('blue')
      | plot([0.3 0 -0.3],[0.5 -0.5 0.5])
  Ypdp : Subsystem  Tag=PSATblock  Description=OPF & CPF  mask(Ypdp){p204q=winter_week_day, p205q=monday, p206q=1, p1x24q=[67 63 60 59 59 60 74 86 95 96 96 95 95 95 93 94 99 100 100 96 91 83 73 63], p25x48q=[78 72 68 66 64 65 66 70 80 88 90 91 90 88 87 87 91 100 99 97 94 92 87 81], p49x72q=[64 60 58 56 56 58 64 76 87 95 99 100 99 100 100 97 96 96 93 92 92 93 87 72], p73x96q=[74 70 66 65 64 62 62 66 81 86 91 93 93 92 91 91 92 94 95 95 100 93 88 80], p97x120q=[63 62 60 58 59 65 72 85 95 99 100 99 93 92 90 88 90 92 96 98 96 90 80 70], p121x144q=[75 73 69 66 65 65 68 74 83 89 92 94 91 90 90 86 85 88 92 100 97 95 90 85], p145x151q=[93 100 98 96 94 77 75], p152x164q=[86 90 87 83 88 84 83 80 74 73 71 72 70], p165x177q=[75 72 80 75 83 87 88 85 81 90 88 89 86], p178x190q=[75 81 80 88 72 77 80 72 72 70 78 69 72], p191x203q=[72 74 74 80 88 88 90 94 89 94 97 100 95]}
      mask prompts: p204q "Select Day Type:"; p205q "Select Day of the Week:"; p206q "Se"; p1x24q "Mask Parameter 4:"; p25x48q "Mask Parameter 5:"; p49x72q "Mask Parameter 6:"; p73x96q "Mask Parameter 7:"; p97x120q "Mask Parameter 8:"; p121x144q "Mask Parameter 9:"; p145x151q "Mask Parameter 10:"; p152x164q "Mask Parameter 11:"; p165x177q "Mask Parameter 12:"; p178x190q "Mask Parameter 13:"; p191x203q "Mask Parameter 14:"
      mask help: This block defines the yearly power demand profile.
      mask TypeOptions p204q: winter_week_day | winter_week_end | summer_week_day | summer_week_end | spring_fall_week_day | spring_fall_week_end
      mask TypeOptions p205q: monday | tuesday | wednesday | thursday | friday | saturday | sunday
      mask Display:
      | plot([-2 22 22 -2 -2],[-1.1 -1.1 1.1 1.1 -1.1])
      | color('blue')
      | plot([0 0 20],[0.8 -0.8 -0.8])
      | color('red')
      | plot([0:19],[ 0.3941  0.5030   0.7220   0.3062   0.1122   0.4433   0.4668   0.0147   0.6641   0.7241   0.2816   0.2618   0.7085   0.7839   0.9862   0.4733   0.9028   0.4511   0.8045   0.8289]-0.2)
      | text(13,-0.25,'Fixed')
  Ypdp1 : Subsystem  Tag=PSATblock  Description=OPF & CPF  mask(Ypdp){pxq=[60 80 100 120 100]}
      mask prompts: pxq "Percentage of load [%]"
      mask help: This block defines the power demand profile (custom length).
      mask Display:
      | plot([-2 22 22 -2 -2],[-1.1 -1.1 1.1 1.1 -1.1])
      | color('blue')
      | plot([0 20],[-0.8 -0.8],[0 0],[-0.8 0.8])
      | color('red')
      | plot([0:19],[ 0.3941  0.5030   0.7220   0.3062   0.1122   0.4433   0.4668   0.0147   0.6641   0.7241   0.2816   0.2618   0.7085   0.7839   0.9862   0.4733   0.9028   0.4511   0.8045   0.8289]-0.2)
      | text(10,-0.25,'Custom')
